simulink model "NLsimWithControllers"  (R2021a)
settings: Solver=ode4  StartTime=0.0  StopTime=30*60  FixedStep=0.01  RelTol=1e-3
undefined symbols (not defined in the file): Earth, sigbuilder_block, WD0, WGS84, X0
libraries: simulink_extras x2, aerolibfltsims x2, aerolibtransform2 x1
settings Model: Creator=User01  LastModifiedBy=User01

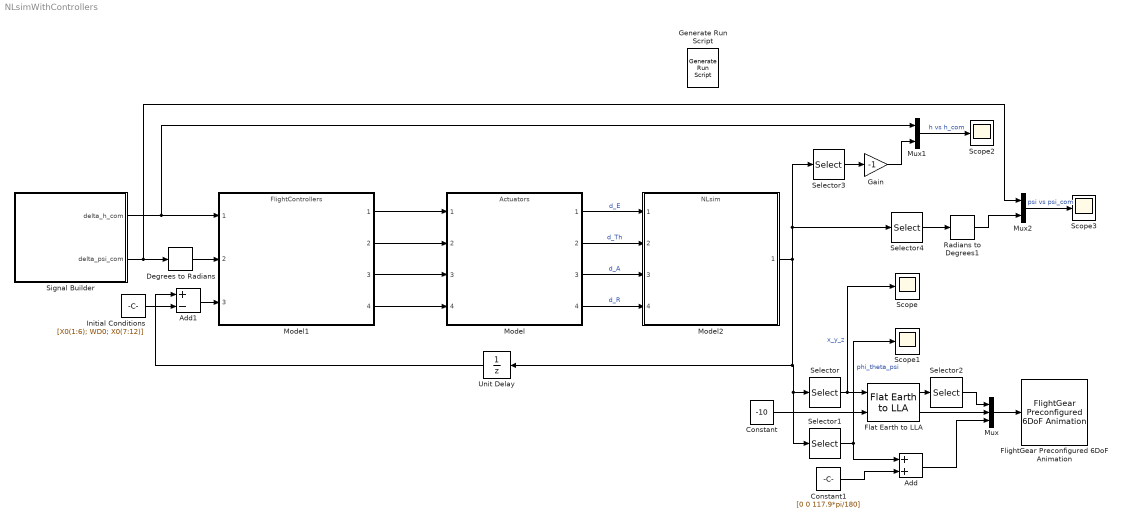
== system NLsimWithControllers ==
  Add : Sum
  Add1 : Sum  Inputs=+-
  Constant : Constant  Value=-10
  Constant1 : Constant  Value=[0 0 117.9*pi/180]
  Degrees to Radians : simulink_extras/Transformations/Degrees to Radians
  Flat Earth to LLA : aerolibtransform2/Flat Earth to LLA  units=English  ptype=Earth (WGS84)  F=1/298.257223563  R=20925646.3255  refPosPort=off  LL0=[37.6285 -122.393]  psi=117.9
  FlightGear Preconfigured 6DoF Animation : aerolibfltsims/FlightGear Preconfigured 6DoF Animation  xFlightGearVersion=v2019.1  DestinationIpAddress=127.0.0.1  DestinationPort=5502  SampleTime=-1  packetVersion=24
  Gain : Gain  Gain=-1
  Generate Run Script : aerolibfltsims/Generate Run Script  Architecture=Win64  dataFlow=Send  GeometryModelName=747-400  AirportId=KSFO  RunwayId=10L  InitialAltitude=7224  InitialHeading=113  OffsetDistance=4.72  OffsetAzimuth=0  InstallScenery=off  DisableShaders=off  OriginAddress=127.0.0.1  DestinationPort=5502  OriginPort=5505  LocalAddress=127.0.0.1  OutputFileName=runfg.bat  FlightGearBaseDirectory=C:\Program Files\FlightGear
  Initial Conditions : Constant  Value=[X0(1:6); WD0; X0(7:12)]
  Model : ModelReference  ModelNameDialog=Actuators.slx  SimulationMode=Normal  ModelReferenceVersion=1.3
  Model1 : ModelReference  ModelNameDialog=FlightControllers.slx  SimulationMode=Normal  ModelReferenceVersion=1.15
  Model2 : ModelReference  ModelNameDialog=NLsim.slx  SimulationMode=Normal  ModelReferenceVersion=1.11
  Mux : Mux  Inputs=3
  Mux1 : Mux  Inputs=2
  Mux2 : Mux  Inputs=2
  Radians to Degrees1 : simulink_extras/Transformations/Radians to Degrees
  Scope{,1..3} (4 alike) : Scope
  Selector : Selector  InputPortWidth=13  IndexOptions=Index vector (dialog)  Indices=[11 12 13]  OutputSizes=1
  Selector1 : Selector  InputPortWidth=13  IndexOptions=Index vector (dialog)  Indices=[8 9 10]  OutputSizes=1
  Selector2 : Selector  InputPortWidth=2  IndexOptions=Index vector (dialog)  Indices=[2 1]  OutputSizes=1
  Selector3 : Selector  InputPortWidth=13  IndexOptions=Index vector (dialog)  Indices=13  OutputSizes=1
  Selector4 : Selector  InputPortWidth=13  IndexOptions=Index vector (dialog)  Indices=10  OutputSizes=1
  Signal Builder : Subsystem  Tag=STV Subsys  LoadFcn=sigbuilder_block('load');  StartFcn=sigbuilder_block('start');  StopFcn=sigbuilder_block('stop');  ClipboardFcn=sigbuilder_block('clipboard');  mask(Sigbuilder block){tuvar=[0:10]}
      mask help: Simulink:masks:SigbuilderBlock_MD
      mask init:
      | if ~strcmp(get_param(bdroot(gcbh),'SimulationStatus'),'stopped') tuvar = sigbuilder_block('maskInit'); end
      settings: CopyFcn=sigbuilder_block('copy');  DeleteFcn=sigbuilder_block('delete');  ModelCloseFcn=sigbuilder_block('modelClose');  PreSaveFcn=sigbuilder_block('preSave');  PauseFcn=sigbuilder_block('pause');  ContinueFcn=sigbuilder_block('continue');  NameChangeFcn=sigbuilder_block('namechange');  OpenFcn=sigbuilder_block('open',[69.75 126.75 550.5 359.25 ]);  CloseFcn=sigbuilder_block('close');
      mask Display: plot(0, 0, 100, 100,[2, 2, 32, 32, 2], [68, 8, 8, 68, 68],[32, 2], [38, 38], [32, 19, 2],[53, 60, 44], [32, 17, 17, 2],[16, 16, 31, 31]);txt = getActiveGroup(gcbh);text(2, 100, txt,'verticalAlignment', 'top');
  Unit Delay : UnitDelay  InitialCondition=[X0(1:6); WD0; X0(7:12)]  SampleTime=-1  HasFrameUpgradeWarning=on
  wires:
  Model1/1 -> Model/1
  Model1/2 -> Model/2
  Model1/3 -> Model/3
  Model1/4 -> Model/4
  Model2/1 -> Selector3/1, Selector4/1, Unit Delay/1, Selector1/1, Selector/1
  Unit Delay/1 -> Add1/1
  Degrees to Radians/1 -> Model1/2
  Initial Conditions/1 -> Add1/2
  Add1/1 -> Model1/3
  Model/1 -> Model2/1  "d_E"
  Model/2 -> Model2/2  "d_Th"
  Model/3 -> Model2/3  "d_A"
  Model/4 -> Model2/4  "d_R"
  Signal Builder/1(delta_h_com) -> Mux1/1, Model1/1
  Selector/1 -> Scope/1, Flat Earth to LLA/1  "x_y_z"
  Flat Earth to LLA/1 -> Selector2/1
  Flat Earth to LLA/2 -> Mux/2
  Selector1/1 -> Add/1, Scope1/1  "phi_theta_psi"
  Mux/1 -> FlightGear Preconfigured 6DoF Animation/1
  Selector2/1 -> Mux/1
  Selector3/1 -> Gain/1
  Gain/1 -> Mux1/2
  Mux1/1 -> Scope2/1  "h vs h_com"
  Mux2/1 -> Scope3/1  "psi vs psi_com"
  Selector4/1 -> Radians to Degrees1/1
  Radians to Degrees1/1 -> Mux2/2
  Signal Builder/2(delta_psi_com) -> Mux2/1, Degrees to Radians/1
  Constant/1 -> Flat Earth to LLA/2
  Add/1 -> Mux/3
  Constant1/1 -> Add/2

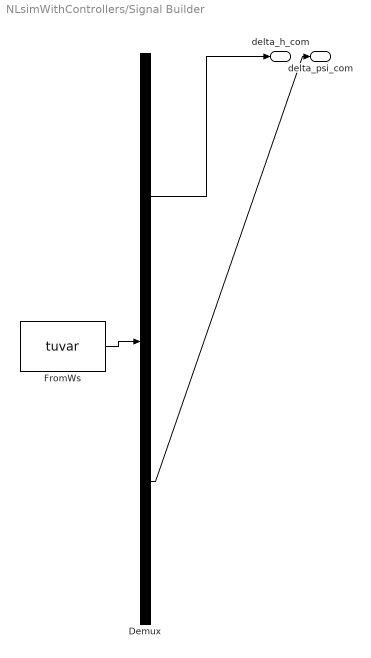
== system NLsimWithControllers/Signal Builder ==
  Demux : Demux  Tag=STV Demux  Outputs=2
      settings: DisplayOption=none
  FromWs : FromWorkspace  Tag=STV FromWs  VariableName=tuvar
      SigBuilderData=|
      | common.afterFinalStr = 'Extrapolate'
      | common.sampleTime = 0
      | dataSet.timeRange = [0 1800]
      | dataSet.name = 'Group 1'
      | sbobj.Groups.Name = 'Group 1'
      | sbobj.Groups.Signals(1).Name = 'delta_h_com'
      | sbobj.Groups.Signals(1).XData = [0 600 1080 1080 1200 1800]
      | sbobj.Groups.Signals(1).YData = [0 10000 10000 10100 10100 0]
      | sbobj.Groups.Signals(2).Name = 'delta_psi_com'
      | sbobj.Groups.Signals(2).XData = [0 720 720 1080 1080 1800]
      | sbobj.Groups.Signals(2).YData = [0 0 360 360 390 390]
      | sbobj.Groups.TimeRange = [0 1800]
  delta_h_com : Outport  Tag=STV Outport
  delta_psi_com : Outport  Tag=STV Outport  Port=2
  wires:
  Demux/1 -> delta_h_com/1
  FromWs/1 -> Demux/1
  Demux/2 -> delta_psi_com/1
